simulink model "hummer_linearized_R2018a"  (R2020b)
settings: Solver=VariableStepAuto  StartTime=0.0  StopTime=10*60  RelTol=1e-3
settings Model: Creator=kjartan  LastModifiedBy=kjartan
settings DebuggingCC: ArithmeticOperatorsInVariantConditions=warning
settings SFSimCC: CustomCodeUndefinedFunction=UseInterfaceOnly

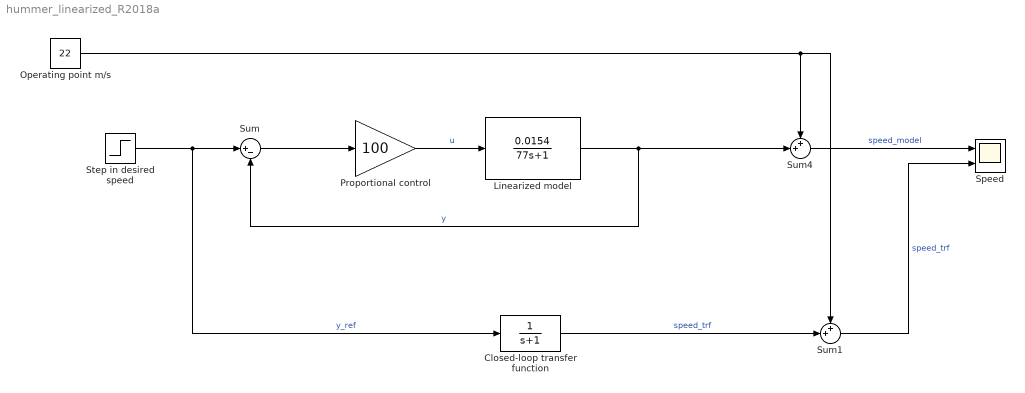
== system hummer_linearized_R2018a ==
  Closed-loop transfer function : TransferFcn  Denominator=[1 1]
  Linearized model : TransferFcn  Numerator=[0.0154]  Denominator=[77 1]
  Operating point m/s : Constant  Value=22
  Proportional control : Gain  Gain=100
  Speed : Scope  NumInputPorts=2
  Step in desired speed : Step  Time=2  After=2  SampleTime=0
  Sum : Sum  Inputs=|+-
  Sum1 : Sum  Inputs=++|
  Sum4 : Sum  Inputs=++|
  wires:
  Sum4/1 -> Speed/1  "speed_model"
  Linearized model/1 -> Sum/2, Sum4/2  "y"
  Operating point m/s/1 -> Sum1/1, Sum4/1
  Proportional control/1 -> Linearized model/1  "u"
  Step in desired speed/1 -> Closed-loop transfer function/1, Sum/1  "y_ref"
  Sum/1 -> Proportional control/1
  Sum1/1 -> Speed/2  "speed_trf"
  Closed-loop transfer function/1 -> Sum1/2  "speed_trf"
